simulink model "LQRsim"  (R2024a)
settings: Solver=VariableStepAuto  StartTime=0.0  StopTime=5  RelTol=1e-3
values from neighbouring files (symbols this model uses):
  A = [0 1;-0.00012 -65.45]    [LQR.m]
  B = [0 ; 44.05]    [LQR.m]
  C = [1 0]    [LQR.m]
  K = place(A,B,p)    [LQR.m]
  Klqr = lqr(sysol,Q,R)    [LQR.m]
  Kr = (1/stepin.Peak)    [LQR.m]
  Krlqr = (1/stepinn.Peak)    [LQR.m]
settings Model: Creator=mingyangpan  LastModifiedBy=mingyangpan

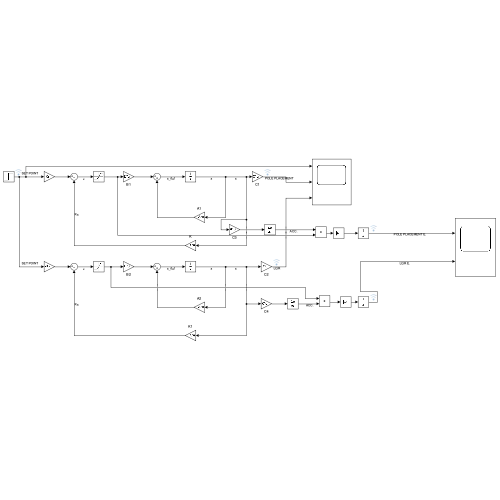
[thumbnail: Simulink's stored preview of the top-level diagram]
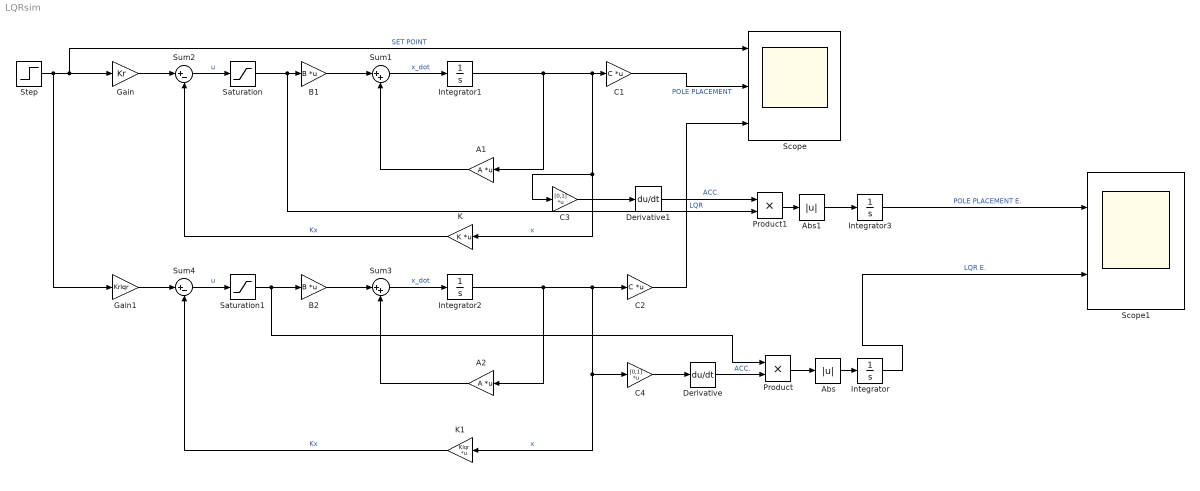
== system LQRsim ==
  A1 : Gain  Gain=A  Multiplication=Matrix(K*u)
  A2 : Gain  Gain=A  Multiplication=Matrix(K*u)
  Abs : Abs  SaturateOnIntegerOverflow=off
  Abs1 : Abs  SaturateOnIntegerOverflow=off
  B1 : Gain  Gain=B  Multiplication=Matrix(K*u)
  B2 : Gain  Gain=B  Multiplication=Matrix(K*u)
  C1 : Gain  Gain=C  Multiplication=Matrix(K*u)
  C2 : Gain  Gain=C  Multiplication=Matrix(K*u)
  C3 : Gain  Gain=[0,1]  Multiplication=Matrix(K*u)
  C4 : Gain  Gain=[0,1]  Multiplication=Matrix(K*u)
  Derivative : Derivative
  Derivative1 : Derivative
  Gain : Gain  Gain=Kr
  Gain1 : Gain  Gain=Krlqr
  Integrator{,1..3} (4 alike) : Integrator
  K : Gain  Gain=K  Multiplication=Matrix(K*u)
  K1 : Gain  Gain=Klqr  Multiplication=Matrix(K*u)
  Product : Product
  Product1 : Product
  Saturation : Saturate  UpperLimit=300  LowerLimit=-300
  Saturation1 : Saturate  UpperLimit=300  LowerLimit=-300
  Scope : Scope  NumInputPorts=3
  Scope1 : Scope  NumInputPorts=2
  Step : Step  SampleTime=0
  Sum1 : Sum  Inputs=|++
  Sum2 : Sum  Inputs=|+-
  Sum3 : Sum  Inputs=|++
  Sum4 : Sum  Inputs=|+-
  wires:
  B1/1 -> Sum1/1
  Sum1/1 -> Integrator1/1  "x_dot"
  Integrator1/1 -> K/1, C3/1, C1/1, A1/1  "x"
  Sum2/1 -> Saturation/1  "u"
  A1/1 -> Sum1/2
  K/1 -> Sum2/2  "Kx"
  Gain/1 -> Sum2/1
  B2/1 -> Sum3/1
  Sum4/1 -> Saturation1/1  "u"
  Integrator2/1 -> C4/1, K1/1, C2/1, A2/1  "x"
  C2/1 -> Scope/3  "LQR"
  A2/1 -> Sum3/2
  Sum3/1 -> Integrator2/1  "x_dot"
  Step/1 -> Gain1/1, Scope/1, Gain/1  "SET POINT"
  Gain1/1 -> Sum4/1
  K1/1 -> Sum4/2  "Kx"
  C1/1 -> Scope/2  "POLE PLACEMENT"
  Saturation/1 -> Product1/2, B1/1
  Saturation1/1 -> Product/1, B2/1
  Derivative1/1 -> Product1/1  "ACC."
  Derivative/1 -> Product/2  "ACC."
  C3/1 -> Derivative1/1
  C4/1 -> Derivative/1
  Product/1 -> Abs/1
  Product1/1 -> Abs1/1
  Abs/1 -> Integrator/1
  Integrator/1 -> Scope1/2  "LQR E."
  Abs1/1 -> Integrator3/1
  Integrator3/1 -> Scope1/1  "POLE PLACEMENT E."
